simulink model "modelMatlabR2019b"  (R2019b)
settings: Solver=ode5  StartTime=0.0  StopTime=settings.Tsim  FixedStep=0.1  RelTol=1e-3
values from neighbouring files (symbols this model uses):
  settings = Simulink.Parameter    [main.m]
settings Model: Creator=rosat  LastModifiedBy=rosat
settings OptimizationCC: BlockReduction=off  DefaultParameterBehavior=Inlined  BufferReuse=off
settings DebuggingCC: SFMachineParentedDataDiag=error

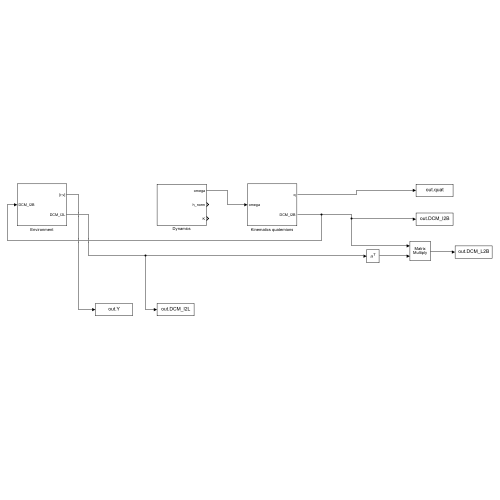
[thumbnail: Simulink's stored preview of the top-level diagram]
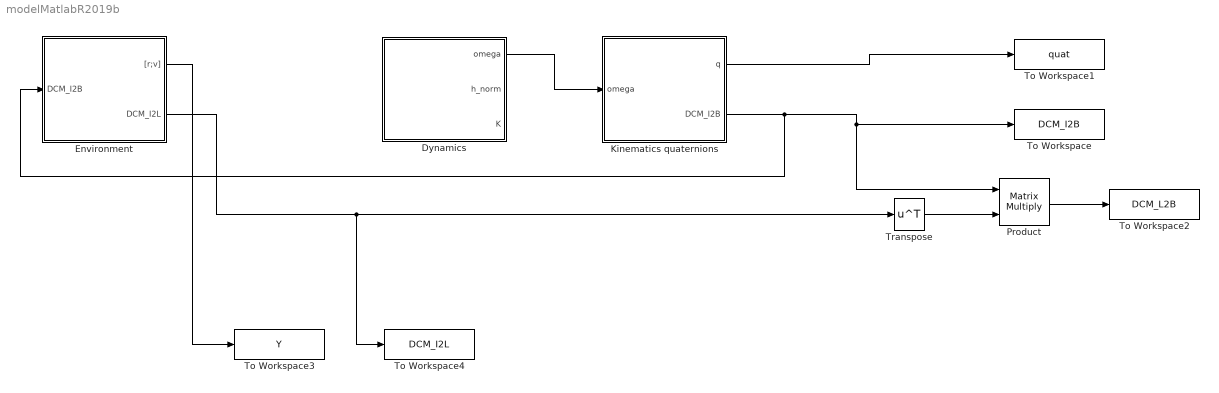
== system modelMatlabR2019b ==
  Dynamics : Subsystem
  Environment : Subsystem
  Kinematics quaternions : Subsystem
  Product : Product  Multiplication=Matrix(*)
  To Workspace : ToWorkspace  VariableName=DCM_I2B  SaveFormat=Timeseries  SampleTime=-1
  To Workspace1 : ToWorkspace  VariableName=quat  SaveFormat=Timeseries  SampleTime=-1
  To Workspace2 : ToWorkspace  VariableName=DCM_L2B  SaveFormat=Timeseries  SampleTime=-1
  To Workspace3 : ToWorkspace  VariableName=Y  SaveFormat=Timeseries  SampleTime=-1
  To Workspace4 : ToWorkspace  VariableName=DCM_I2L  SaveFormat=Timeseries  SampleTime=-1
  Transpose : Math  Operator=transpose  SaturateOnIntegerOverflow=on
  wires:
  Dynamics/1(omega) -> Kinematics quaternions/1(omega)
  Kinematics quaternions/2(DCM_I2B) -> Environment/1(DCM_I2B), To Workspace/1, Product/1
  Kinematics quaternions/1(q) -> To Workspace1/1
  Environment/2(DCM_I2L) -> To Workspace4/1, Transpose/1
  Transpose/1 -> Product/2
  Product/1 -> To Workspace2/1
  Environment/1("[r;v]") -> To Workspace3/1

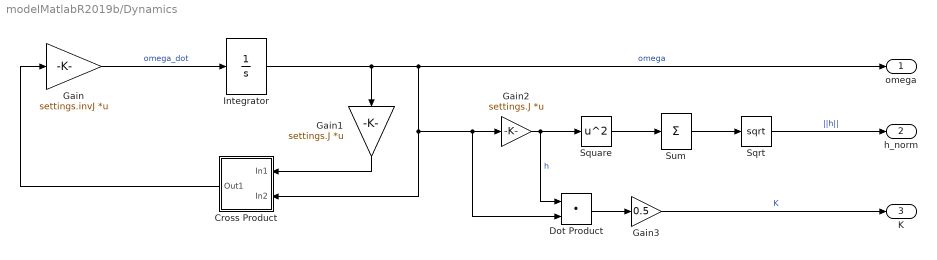
== system modelMatlabR2019b/Dynamics ==
  Cross Product : Subsystem  Description=Replaced Block  mask(Replaced Block){}
      mask help: This block has been replaced with an empty subsystem because it used functionality that is unavailable in Simulink R2019b.
      mask Display: fprintf('Replaced: %s\n','CrossProduct')
  Dot Product : DotProduct  InputSameDT=on  OutDataTypeStr=Inherit: Inherit via internal rule
  Gain : Gain  Gain=settings.invJ  Multiplication=Matrix(K*u)
  Gain1 : Gain  Gain=settings.J  Multiplication=Matrix(K*u)
  Gain2 : Gain  Gain=settings.J  Multiplication=Matrix(K*u)
  Gain3 : Gain  Gain=0.5
  Integrator : Integrator  InitialCondition=settings.omega0
  Sqrt : Sqrt  SaturateOnIntegerOverflow=on
  Square : Math  Operator=square  SaturateOnIntegerOverflow=on
  Sum : Sum  Inputs=+
  omega : Outport
  h_norm : Outport  Port=2
  K : Outport  Port=3
  wires:
  Sqrt/1 -> h_norm/1  "||h||"
  Gain3/1 -> K/1  "K"
  Gain/1 -> Integrator/1  "omega_dot"
  Integrator/1 -> Gain1/1, Dot Product/2, Gain2/1, Cross Product/2(In2), omega/1  "omega"
  Gain2/1 -> Square/1, Dot Product/1  "h"
  Cross Product/1(Out1) -> Gain/1
  Gain1/1 -> Cross Product/1(In1)
  Dot Product/1 -> Gain3/1
  Square/1 -> Sum/1
  Sum/1 -> Sqrt/1

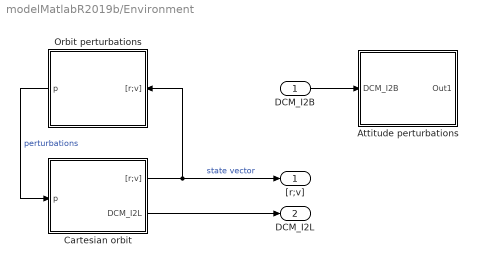
== system modelMatlabR2019b/Environment ==
  DCM_I2B : Inport
  Attitude perturbations : Subsystem
  Cartesian orbit : Subsystem
  Orbit perturbations : Subsystem
  "[r;v]" : Outport
  DCM_I2L : Outport  Port=2
  wires:
  Cartesian orbit/2(DCM_I2L) -> DCM_I2L/1
  Cartesian orbit/1("[r;v]") -> Orbit perturbations/1("[r;v]"), "[r;v]"/1  "state vector"
  Orbit perturbations/1(p) -> Cartesian orbit/1(p)  "perturbations"
  DCM_I2B/1 -> Attitude perturbations/1(DCM_I2B)

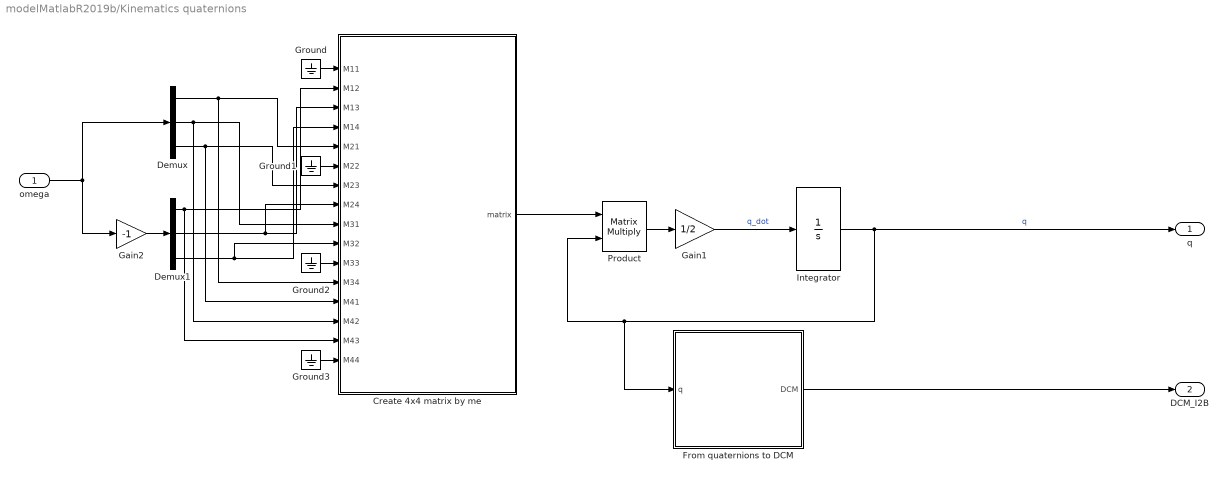
== system modelMatlabR2019b/Kinematics quaternions ==
  omega : Inport
  Create 4x4 matrix by me : Subsystem
  Demux : Demux  Outputs=3
  Demux1 : Demux  Outputs=3
  From quaternions to DCM : Subsystem
  Gain1 : Gain  Gain=1/2
  Gain2 : Gain  Gain=-1
  Ground{,1..3} (4 alike) : Ground
  Integrator : Integrator  InitialCondition=settings.q0
  Product : Product  Multiplication=Matrix(*)
  q : Outport
  DCM_I2B : Outport  Port=2
  wires:
  omega/1 -> Demux/1, Gain2/1
  Ground/1 -> Create 4x4 matrix by me/1(M11)
  Ground1/1 -> Create 4x4 matrix by me/6(M22)
  Ground2/1 -> Create 4x4 matrix by me/11(M33)
  Ground3/1 -> Create 4x4 matrix by me/16(M44)
  Gain1/1 -> Integrator/1  "q_dot"
  Integrator/1 -> q/1, From quaternions to DCM/1(q), Product/2  "q"
  Product/1 -> Gain1/1
  Create 4x4 matrix by me/1(matrix) -> Product/1
  From quaternions to DCM/1(DCM) -> DCM_I2B/1
  Demux1/1 -> Create 4x4 matrix by me/15(M43), Create 4x4 matrix by me/2(M12)
  Demux1/2 -> Create 4x4 matrix by me/8(M24), Create 4x4 matrix by me/3(M13)
  Demux1/3 -> Create 4x4 matrix by me/10(M32), Create 4x4 matrix by me/4(M14)
  Demux/1 -> Create 4x4 matrix by me/12(M34), Create 4x4 matrix by me/5(M21)
  Demux/3 -> Create 4x4 matrix by me/13(M41), Create 4x4 matrix by me/7(M23)
  Demux/2 -> Create 4x4 matrix by me/14(M42), Create 4x4 matrix by me/9(M31)
  Gain2/1 -> Demux1/1

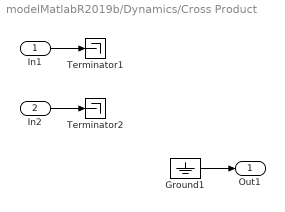
== system modelMatlabR2019b/Dynamics/Cross Product ==
  In1 : Inport
  In2 : Inport  Port=2
  Ground1 : Ground
  Terminator1 : Terminator
  Terminator2 : Terminator
  Out1 : Outport
  wires:
  Ground1/1 -> Out1/1
  In2/1 -> Terminator2/1
  In1/1 -> Terminator1/1

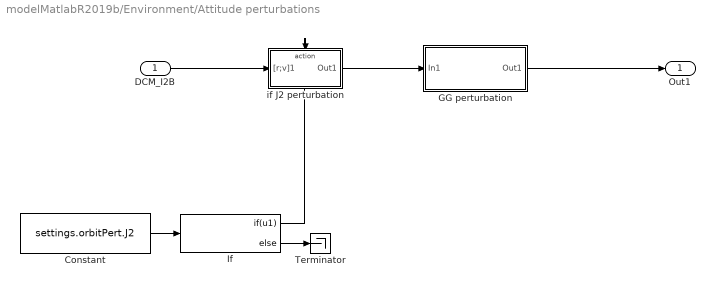
== system modelMatlabR2019b/Environment/Attitude perturbations ==
  DCM_I2B : Inport
  Constant : Constant  Value=settings.orbitPert.J2
  GG perturbation : Subsystem
  If : If  IfExpression=u1
  Terminator : Terminator
  if J2 perturbation : Subsystem  TreatAsAtomicUnit=on
  Out1 : Outport
  wires:
  DCM_I2B/1 -> if J2 perturbation/1("[r;v]1")
  If/1 -> if J2 perturbation/Action
  If/2 -> Terminator/1
  Constant/1 -> If/1
  if J2 perturbation/1(Out1) -> GG perturbation/1(In1)
  GG perturbation/1(Out1) -> Out1/1

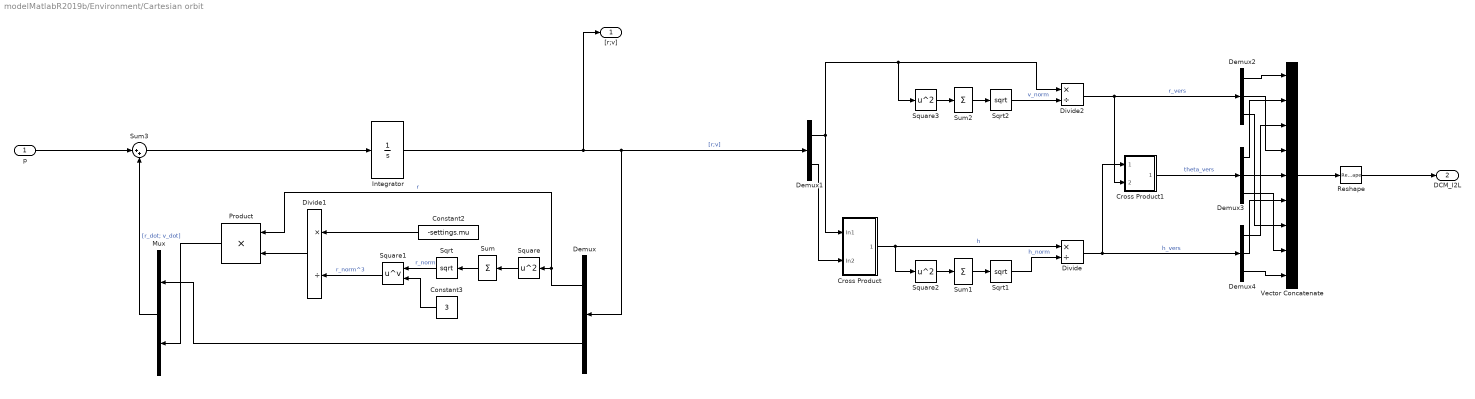
== system modelMatlabR2019b/Environment/Cartesian orbit ==
  p : Inport
  Constant2 : Constant  Value=-settings.mu
  Constant3 : Constant  Value=3
  Cross Product : Subsystem  Description=Replaced Block  mask(Replaced Block){}
      mask help: This block has been replaced with an empty subsystem because it used functionality that is unavailable in Simulink R2019b.
      mask Display: fprintf('Replaced: %s\n','CrossProduct')
  Cross Product1 : Subsystem  Description=Replaced Block  mask(Replaced Block){}
      mask help: This block has been replaced with an empty subsystem because it used functionality that is unavailable in Simulink R2019b.
      mask Display: fprintf('Replaced: %s\n','CrossProduct')
  Demux : Demux  Outputs=2
  Demux1 : Demux  Outputs=2
  Demux2 : Demux  Outputs=3
  Demux3 : Demux  Outputs=3
  Demux4 : Demux  Outputs=3
  Divide : Product  Inputs=*/
  Divide1 : Product  Inputs=*/
  Divide2 : Product  Inputs=*/
  Integrator : Integrator  InitialCondition=settings.Y0
  Mux : Mux  Inputs=2
  Product : Product
  Reshape : Reshape  OutputDimensionality=Customize  OutputDimensions=[3,3]
  Sqrt : Sqrt  SaturateOnIntegerOverflow=on
  Sqrt1 : Sqrt  SaturateOnIntegerOverflow=on
  Sqrt2 : Sqrt  SaturateOnIntegerOverflow=on
  Square : Math  Operator=square  SaturateOnIntegerOverflow=on
  Square1 : Math  Operator=pow  SaturateOnIntegerOverflow=on
  Square2 : Math  Operator=square  SaturateOnIntegerOverflow=on
  Square3 : Math  Operator=square  SaturateOnIntegerOverflow=on
  Sum : Sum  Inputs=+
  Sum1 : Sum  Inputs=+
  Sum2 : Sum  Inputs=+
  Sum3 : Sum  Inputs=|++
  Vector Concatenate : Concatenate  NumInputs=9
  "[r;v]" : Outport
  DCM_I2L : Outport  Port=2
  wires:
  Constant3/1 -> Square1/2
  Demux/1 -> Product/1, Square/1  "r"
  Demux/2 -> Mux/1
  Integrator/1 -> Demux1/1, Demux/1, "[r;v]"/1  "[r;v]"
  Divide1/1 -> Product/2
  Sqrt/1 -> Square1/1  "r_norm"
  Constant2/1 -> Divide1/1
  Product/1 -> Mux/2
  Sum/1 -> Sqrt/1
  Square/1 -> Sum/1
  Square1/1 -> Divide1/2  "r_norm^3"
  Mux/1 -> Sum3/2  "[r_dot; v_dot]"
  Sqrt2/1 -> Divide2/2  "v_norm"
  Divide2/1 -> Cross Product1/2(In2), Demux2/1  "r_vers"
  Demux1/1 -> Square3/1, Divide2/1, Cross Product/1(In1)
  Demux2/2 -> Vector Concatenate/4
  Sqrt1/1 -> Divide/2  "h_norm"
  Demux4/1 -> Vector Concatenate/3
  Demux4/3 -> Vector Concatenate/9
  Demux3/3 -> Vector Concatenate/8
  Demux4/2 -> Vector Concatenate/6
  Vector Concatenate/1 -> Reshape/1
  Divide/1 -> Cross Product1/1(In1), Demux4/1  "h_vers"
  Demux3/1 -> Vector Concatenate/2
  Sum1/1 -> Sqrt1/1
  Demux2/3 -> Vector Concatenate/7
  Square2/1 -> Sum1/1
  Demux2/1 -> Vector Concatenate/1
  Demux3/2 -> Vector Concatenate/5
  Cross Product/1(Out1) -> Divide/1, Square2/1  "h"
  Square3/1 -> Sum2/1
  Sum2/1 -> Sqrt2/1
  Cross Product1/1(Out1) -> Demux3/1  "theta_vers"
  Reshape/1 -> DCM_I2L/1
  Demux1/2 -> Cross Product/2(In2)
  Sum3/1 -> Integrator/1
  p/1 -> Sum3/1

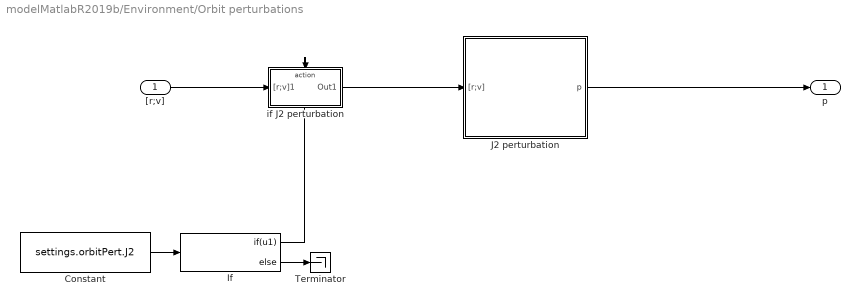
== system modelMatlabR2019b/Environment/Orbit perturbations ==
  "[r;v]" : Inport
  Constant : Constant  Value=settings.orbitPert.J2
  If : If  IfExpression=u1
  J2 perturbation : Subsystem
  Terminator : Terminator
  if J2 perturbation : Subsystem  TreatAsAtomicUnit=on
  p : Outport
  wires:
  "[r;v]"/1 -> if J2 perturbation/1("[r;v]1")
  if J2 perturbation/1(Out1) -> J2 perturbation/1("[r;v]")
  J2 perturbation/1(p) -> p/1
  Constant/1 -> If/1
  If/2 -> Terminator/1
  If/1 -> if J2 perturbation/Action

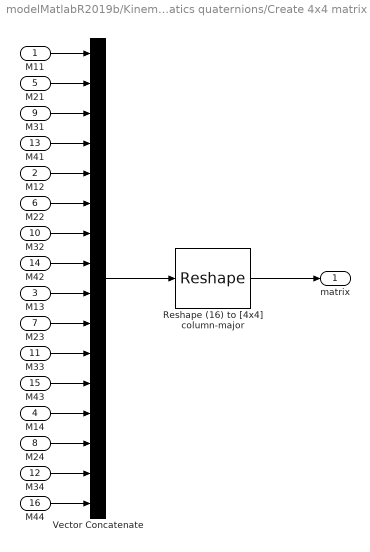
== system modelMatlabR2019b/Kinematics quaternions/Create 4x4 matrix by me ==
  M11 : Inport
  M12 : Inport  Port=2
  M13 : Inport  Port=3
  M14 : Inport  Port=4
  M21 : Inport  Port=5
  M22 : Inport  Port=6
  M23 : Inport  Port=7
  M24 : Inport  Port=8
  M31 : Inport  Port=9
  M32 : Inport  Port=10
  M33 : Inport  Port=11
  M34 : Inport  Port=12
  M41 : Inport  Port=13
  M42 : Inport  Port=14
  M43 : Inport  Port=15
  M44 : Inport  Port=16
  Reshape (16) to [4x4] column-major : Reshape  OutputDimensionality=Customize  OutputDimensions=[4,4]
  Vector Concatenate : Concatenate  NumInputs=16
  matrix : Outport
  wires:
  M12/1 -> Vector Concatenate/5
  M11/1 -> Vector Concatenate/1
  M13/1 -> Vector Concatenate/9
  M14/1 -> Vector Concatenate/13
  M21/1 -> Vector Concatenate/2
  M44/1 -> Vector Concatenate/16
  M34/1 -> Vector Concatenate/15
  M24/1 -> Vector Concatenate/14
  M43/1 -> Vector Concatenate/12
  M33/1 -> Vector Concatenate/11
  M23/1 -> Vector Concatenate/10
  M42/1 -> Vector Concatenate/8
  M32/1 -> Vector Concatenate/7
  M22/1 -> Vector Concatenate/6
  M41/1 -> Vector Concatenate/4
  M31/1 -> Vector Concatenate/3
  Vector Concatenate/1 -> Reshape (16) to [4x4] column-major/1
  Reshape (16) to [4x4] column-major/1 -> matrix/1

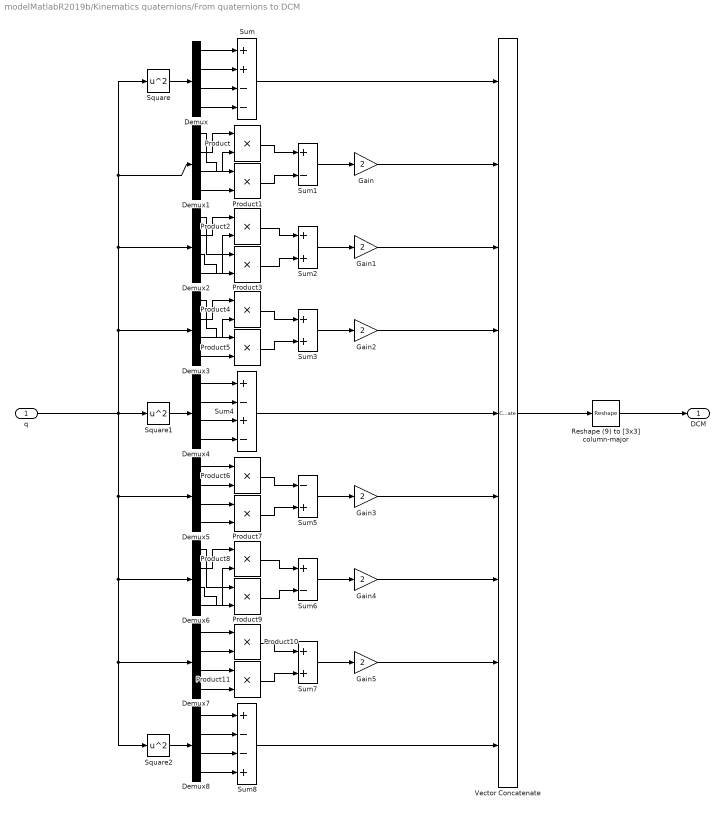
== system modelMatlabR2019b/Kinematics quaternions/From quaternions to DCM ==
  q : Inport
  Demux{,1..8} (9 alike) : Demux
  Gain{,1..5} (6 alike) : Gain  Gain=2
  Product{,1..11} (12 alike) : Product
  Reshape (9) to [3x3] column-major : Reshape  OutputDimensionality=Customize  OutputDimensions=[3,3]
  Square : Math  Operator=square  SaturateOnIntegerOverflow=on
  Square1 : Math  Operator=square  SaturateOnIntegerOverflow=on
  Square2 : Math  Operator=square  SaturateOnIntegerOverflow=on
  Sum : Sum  Inputs=++--
  Sum1 : Sum  Inputs=+-
  Sum2 : Sum
  Sum3 : Sum
  Sum4 : Sum  Inputs=+-+-
  Sum5 : Sum  Inputs=-+
  Sum6 : Sum  Inputs=+-
  Sum7 : Sum
  Sum8 : Sum  Inputs=+--+
  Vector Concatenate : Concatenate  NumInputs=9
  DCM : Outport
  wires:
  q/1 -> Square/1, Demux1/1, Demux2/1, Demux3/1, Square1/1, Demux5/1, Demux6/1, Demux7/1, Square2/1
  Vector Concatenate/1 -> Reshape (9) to [3x3] column-major/1
  Square/1 -> Demux/1
  Demux/3 -> Sum/3
  Demux/4 -> Sum/4
  Demux/2 -> Sum/2
  Demux/1 -> Sum/1
  Sum/1 -> Vector Concatenate/1
  Demux1/2 -> Product/1
  Demux1/3 -> Product/2
  Demux1/1 -> Product1/1
  Demux1/4 -> Product1/2
  Product/1 -> Sum1/1
  Product1/1 -> Sum1/2
  Sum1/1 -> Gain/1
  Gain/1 -> Vector Concatenate/2
  Demux2/2 -> Product2/1
  Demux2/4 -> Product2/2
  Demux2/1 -> Product3/1
  Demux2/3 -> Product3/2
  Product3/1 -> Sum2/2
  Product2/1 -> Sum2/1
  Sum2/1 -> Gain1/1
  Gain1/1 -> Vector Concatenate/3
  Demux3/1 -> Product5/1
  Product5/1 -> Sum3/2
  Demux3/2 -> Product4/1
  Product4/1 -> Sum3/1
  Demux3/3 -> Product4/2
  Demux3/4 -> Product5/2
  Sum3/1 -> Gain2/1
  Gain2/1 -> Vector Concatenate/4
  Demux4/3 -> Sum4/3
  Demux4/1 -> Sum4/1
  Demux4/4 -> Sum4/4
  Sum4/1 -> Vector Concatenate/5
  Demux4/2 -> Sum4/2
  Square1/1 -> Demux4/1
  Product7/1 -> Sum5/2
  Product6/1 -> Sum5/1
  Sum5/1 -> Gain3/1
  Demux5/3 -> Product7/1
  Demux5/4 -> Product7/2
  Demux5/1 -> Product6/1
  Demux5/2 -> Product6/2
  Gain3/1 -> Vector Concatenate/6
  Sum6/1 -> Gain4/1
  Demux6/2 -> Product8/1
  Gain4/1 -> Vector Concatenate/7
  Demux6/4 -> Product8/2
  Demux6/3 -> Product9/2
  Demux6/1 -> Product9/1
  Product9/1 -> Sum6/2
  Product8/1 -> Sum6/1
  Demux7/2 -> Product10/2
  Demux7/3 -> Product11/1
  Sum7/1 -> Gain5/1
  Product10/1 -> Sum7/1
  Demux7/1 -> Product10/1
  Demux7/4 -> Product11/2
  Product11/1 -> Sum7/2
  Gain5/1 -> Vector Concatenate/8
  Demux8/2 -> Sum8/2
  Square2/1 -> Demux8/1
  Sum8/1 -> Vector Concatenate/9
  Demux8/3 -> Sum8/3
  Reshape (9) to [3x3] column-major/1 -> DCM/1
  Demux8/1 -> Sum8/1
  Demux8/4 -> Sum8/4

== system modelMatlabR2019b/Environment/Attitude perturbations/GG perturbation ==
  In1 : Inport
  Out1 : Outport
  wires:
  In1/1 -> Out1/1

== system modelMatlabR2019b/Environment/Attitude perturbations/if J2 perturbation ==
  "[r;v]1" : Inport
  Action Port : ActionPort  ActionPortLabel=if(u1)
  Out1 : Outport
  wires:
  "[r;v]1"/1 -> Out1/1

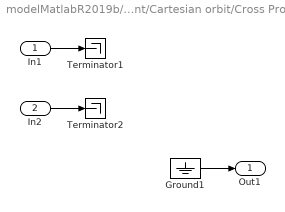
== system modelMatlabR2019b/Environment/Cartesian orbit/Cross Product ==
  In1 : Inport
  In2 : Inport  Port=2
  Ground1 : Ground
  Terminator1 : Terminator
  Terminator2 : Terminator
  Out1 : Outport
  wires:
  Ground1/1 -> Out1/1
  In2/1 -> Terminator2/1
  In1/1 -> Terminator1/1

== system modelMatlabR2019b/Environment/Cartesian orbit/Cross Product1 ==
  In1 : Inport
  In2 : Inport  Port=2
  Ground1 : Ground
  Terminator1 : Terminator
  Terminator2 : Terminator
  Out1 : Outport
  wires:
  Ground1/1 -> Out1/1
  In2/1 -> Terminator2/1
  In1/1 -> Terminator1/1

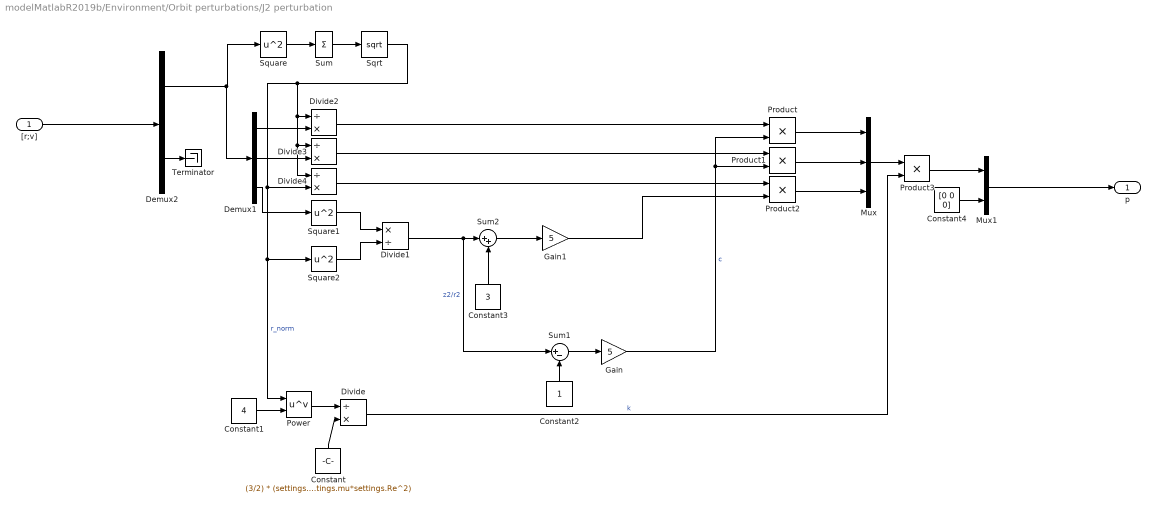
== system modelMatlabR2019b/Environment/Orbit perturbations/J2 perturbation ==
  "[r;v]" : Inport
  Constant : Constant  Value=(3/2) * (settings.orbitPert.J2value*settings.mu*settings.Re^2)
  Constant1 : Constant  Value=4
  Constant2 : Constant
  Constant3 : Constant  Value=3
  Constant4 : Constant  Value=[0 0 0]
  Demux1 : Demux  Outputs=3
  Demux2 : Demux  Outputs=2
  Divide{,2..4} (4 alike) : Product  Inputs=/*
  Divide1 : Product  Inputs=*/
  Gain : Gain  Gain=5
  Gain1 : Gain  Gain=5
  Mux : Mux  Inputs=3
  Mux1 : Mux  Inputs=2
  Power : Math  Operator=pow  SaturateOnIntegerOverflow=on
  Product{,1..3} (4 alike) : Product
  Sqrt : Sqrt  SaturateOnIntegerOverflow=on
  Square : Math  Operator=square  SaturateOnIntegerOverflow=on
  Square1 : Math  Operator=square  SaturateOnIntegerOverflow=on
  Square2 : Math  Operator=square  SaturateOnIntegerOverflow=on
  Sum : Sum  Inputs=+
  Sum1 : Sum  Inputs=|+-
  Sum2 : Sum  Inputs=|++
  Terminator : Terminator
  p : Outport
  wires:
  "[r;v]"/1 -> Demux2/1
  Demux2/2 -> Terminator/1
  Square/1 -> Sum/1
  Sum/1 -> Sqrt/1
  Sqrt/1 -> Divide4/1, Divide3/1, Divide2/1, Divide4/2, Power/1, Square2/1  "r_norm"
  Demux2/1 -> Demux1/1, Square/1
  Constant/1 -> Divide/2
  Constant1/1 -> Power/2
  Power/1 -> Divide/1
  Demux1/3 -> Square1/1
  Square1/1 -> Divide1/1
  Square2/1 -> Divide1/2
  Constant2/1 -> Sum1/2
  Divide1/1 -> Sum1/1, Sum2/1  "z2/r2"
  Sum1/1 -> Gain/1
  Gain/1 -> Product1/2, Product/2  "c"
  Divide/1 -> Product3/2  "k"
  Demux1/1 -> Divide2/2
  Divide2/1 -> Product/1
  Demux1/2 -> Divide3/2
  Divide3/1 -> Product1/1
  Constant3/1 -> Sum2/2
  Sum2/1 -> Gain1/1
  Divide4/1 -> Product2/1
  Gain1/1 -> Product2/2
  Product/1 -> Mux/1
  Product1/1 -> Mux/2
  Product2/1 -> Mux/3
  Mux/1 -> Product3/1
  Product3/1 -> Mux1/1
  Constant4/1 -> Mux1/2
  Mux1/1 -> p/1

== system modelMatlabR2019b/Environment/Orbit perturbations/if J2 perturbation ==
  "[r;v]1" : Inport
  Action Port : ActionPort  ActionPortLabel=if(u1)
  Out1 : Outport
  wires:
  "[r;v]1"/1 -> Out1/1
